simulink subsystem "BypassHouse"  (R2023a)
settings: Solver=VariableStepAuto  StartTime=0.0  StopTime=10.0  RelTol=1e-3
undefined symbols (not defined in the file): A, K
libraries: mpclib x1
settings Model: Creator=giaco  LastModifiedBy=giaco

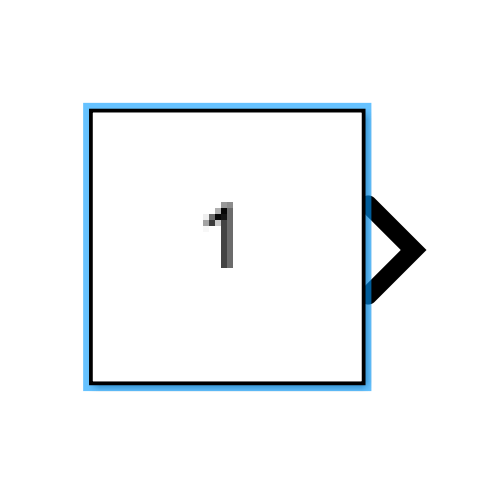
[thumbnail: Simulink's stored preview of the top-level diagram]
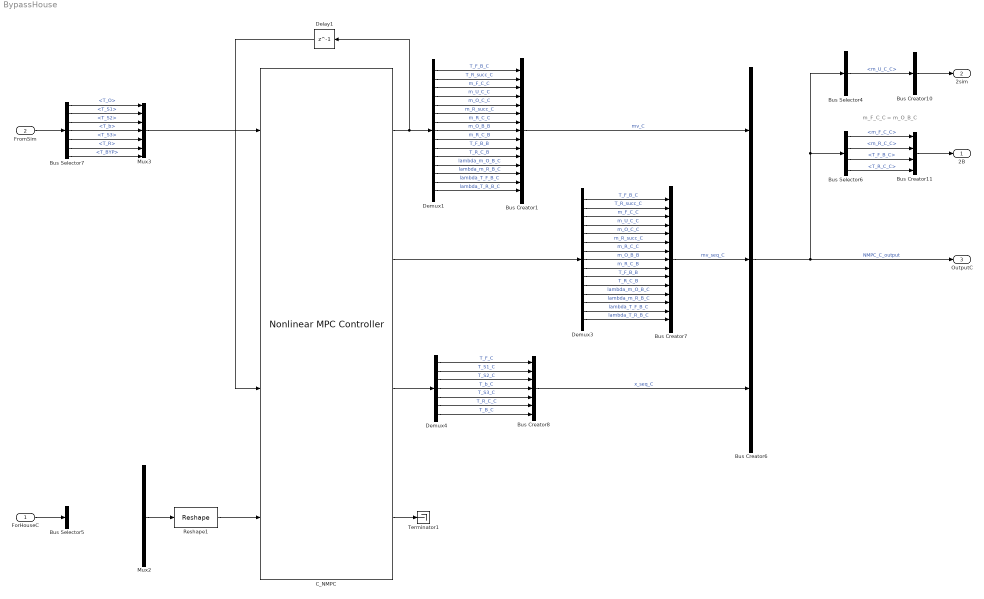
== system BypassHouse ==
  note: m_F_C_C = m_O_B_C
  ForHouseC : Inport
  FromSim : Inport  Port=2
  Bus Creator1 : BusCreator  Inputs=15  OutDataTypeStr=Bus: Bus_mv_C
  Bus Creator10 : BusCreator  Inputs=1
  Bus Creator11 : BusCreator  Inputs=4
  Bus Creator6 : BusCreator  Inputs=3  OutDataTypeStr=Bus: NMPC_C_output
  Bus Creator7 : BusCreator  Inputs=15  OutDataTypeStr=Bus: Bus_mv_seq_C
  Bus Creator8 : BusCreator  Inputs=7  OutDataTypeStr=Bus: Bus_x_seq_C
  Bus Selector4 : BusSelector  OutputSignals=mv_C.m_U_C_C
  Bus Selector5 : BusSelector  OutputSignals=signal1,A_storage
  Bus Selector6 : BusSelector  OutputSignals=mv_seq_C.m_F_C_C,mv_seq_C.m_R_C_C,mv_seq_C.T_F_B_C,x_seq_C.T_R_C_C
  Bus Selector7 : BusSelector  OutputSignals=T_O,T_S1,T_S2,T_b,T_S3,T_R,T_BYP
  C_NMPC : mpclib/Nonlinear MPC Controller  nlmpcobj=C.nlobj  UseObjectTs=on  UseMEX=off  md_enabled=on  mvtarget_enabled=off  param_enabled=off  cost_enabled=off  mvseq_enabled=on  stateseq_enabled=on  ovseq_enabled=off  slack_enabled=off  status_enabled=on  ov_min=off  ov_max=off  mv_min=off  mv_max=off  mvrate_min=off  mvrate_max=off  state_min=off  state_max=off  ov_weight=off  mv_weight=off  mvrate_weight=off  ecr_weight=off  nlp_initialize=off
  Delay1 : Delay  DelayLength=1
  Demux1 : Demux  Outputs=15
  Demux3 : Demux  Outputs=15
  Demux4 : Demux  Outputs=7
  Mux2 : Mux  Inputs=12
  Mux3 : Mux  Inputs=7
  Reshape1 : Reshape  OutputDimensionality=Customize  OutputDimensions=[K,A.nu_md]
  Terminator1 : Terminator
  2B : Outport
  2sim : Outport  Port=2
  OutputC : Outport  Port=3
  wires:
  Demux3/9 -> Bus Creator7/9  "m_R_C_B"
  Demux3/4 -> Bus Creator7/4  "m_U_C_C"
  Demux3/2 -> Bus Creator7/2  "T_R_succ_C"
  Demux3/6 -> Bus Creator7/6  "m_R_succ_C"
  Demux3/3 -> Bus Creator7/3  "m_F_C_C"
  Bus Creator1/1 -> Bus Creator6/1  "mv_C"
  Demux3/11 -> Bus Creator7/11  "T_R_C_B"
  C_NMPC/3 -> Demux4/1
  ForHouseC/1 -> Bus Selector5/1
  FromSim/1 -> Bus Selector7/1
  Mux2/1 -> Reshape1/1
  Demux3/7 -> Bus Creator7/7  "m_R_C_C"
  Bus Creator11/1 -> 2B/1
  Bus Creator10/1 -> 2sim/1
  Demux4/1 -> Bus Creator8/1  "T_F_C"
  Demux4/6 -> Bus Creator8/6  "T_R_C_C"
  Bus Selector6/1 -> Bus Creator11/1  "<m_F_C_C>"
  Demux4/5 -> Bus Creator8/5  "T_S3_C"
  Demux4/3 -> Bus Creator8/3  "T_S2_C"
  Bus Selector6/3 -> Bus Creator11/3  "<T_F_B_C>"
  Demux4/4 -> Bus Creator8/4  "T_b_C"
  Demux3/14 -> Bus Creator7/14  "lambda_T_F_B_C"
  Demux4/2 -> Bus Creator8/2  "T_S1_C"
  Mux3/1 -> C_NMPC/1
  Demux3/5 -> Bus Creator7/5  "m_O_C_C"
  Demux3/8 -> Bus Creator7/8  "m_O_B_B"
  C_NMPC/4 -> Terminator1/1
  Bus Selector6/2 -> Bus Creator11/2  "<m_R_C_C>"
  Demux3/1 -> Bus Creator7/1  "T_F_B_C"
  Bus Creator6/1 -> OutputC/1, Bus Selector6/1, Bus Selector4/1  "NMPC_C_output"
  Bus Selector4/1 -> Bus Creator10/1  "<m_U_C_C>"
  Demux3/13 -> Bus Creator7/13  "lambda_m_R_B_C"
  Delay1/1 -> C_NMPC/3
  Demux3/15 -> Bus Creator7/15  "lambda_T_R_B_C"
  Bus Creator7/1 -> Bus Creator6/2  "mv_seq_C"
  Demux3/10 -> Bus Creator7/10  "T_F_B_B"
  Reshape1/1 -> C_NMPC/4
  Demux3/12 -> Bus Creator7/12  "lambda_m_O_B_C"
  C_NMPC/2 -> Demux3/1
  Bus Creator8/1 -> Bus Creator6/3  "x_seq_C"
  Demux4/7 -> Bus Creator8/7  "T_B_C"
  Demux1/9 -> Bus Creator1/9  "m_R_C_B"
  Demux1/12 -> Bus Creator1/12  "lambda_m_O_B_C"
  Demux1/11 -> Bus Creator1/11  "T_R_C_B"
  Demux1/2 -> Bus Creator1/2  "T_R_succ_C"
  Demux1/3 -> Bus Creator1/3  "m_F_C_C"
  Demux1/15 -> Bus Creator1/15  "lambda_T_R_B_C"
  Demux1/1 -> Bus Creator1/1  "T_F_B_C"
  Demux1/13 -> Bus Creator1/13  "lambda_m_R_B_C"
  Demux1/7 -> Bus Creator1/7  "m_R_C_C"
  Demux1/5 -> Bus Creator1/5  "m_O_C_C"
  Demux1/4 -> Bus Creator1/4  "m_U_C_C"
  Demux1/14 -> Bus Creator1/14  "lambda_T_F_B_C"
  Demux1/6 -> Bus Creator1/6  "m_R_succ_C"
  Demux1/10 -> Bus Creator1/10  "T_F_B_B"
  Demux1/8 -> Bus Creator1/8  "m_O_B_B"
  C_NMPC/1 -> Delay1/1, Demux1/1
  Bus Selector6/4 -> Bus Creator11/4  "<T_R_C_C>"
  Bus Selector7/1 -> Mux3/1  "<T_O>"
  Bus Selector7/2 -> Mux3/2  "<T_S1>"
  Bus Selector7/3 -> Mux3/3  "<T_S2>"
  Bus Selector7/4 -> Mux3/4  "<T_b>"
  Bus Selector7/5 -> Mux3/5  "<T_S3>"
  Bus Selector7/6 -> Mux3/6  "<T_R>"
  Bus Selector7/7 -> Mux3/7  "<T_BYP>"
